simulink model "similinkProj"  (R2016a)
settings: Solver=VariableStepAuto  StartTime=0.0  StopTime=5  RelTol=1e-3
settings Model: Creator=bmcilw1  LastModifiedBy=bmcilw1

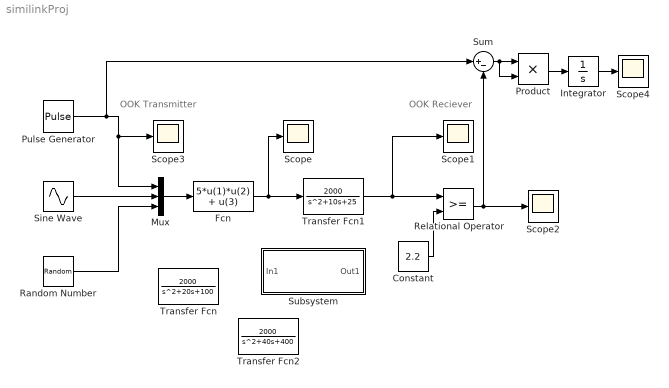
== system similinkProj ==
  note: OOK Transmitter
  note: OOK Reciever
  Constant : Constant  Value=2.2
  Fcn : Fcn  Expr=5*u(1)*u(2) + u(3)
  Integrator : Integrator
  Mux : Mux  Inputs=3
  Product : Product
  Pulse Generator : DiscretePulseGenerator  PulseType=Time based  PulseWidth=10  PhaseDelay=.2
  Random Number : RandomNumber  Variance=.25  SampleTime=0.001
  Relational Operator : RelationalOperator  OutDataTypeStr=boolean
  Scope{,1..4} (5 alike) : Scope
  Sine Wave : Sin  Amplitude=3  Frequency=50*2*pi  SampleTime=0.001
  Subsystem : Subsystem
  Sum : Sum  Inputs=|+-
  Transfer Fcn : TransferFcn  Numerator=[2000]  Denominator=[1 20 100]
  Transfer Fcn1 : TransferFcn  Numerator=[2000]  Denominator=[1 10 25]
  Transfer Fcn2 : TransferFcn  Numerator=[2000]  Denominator=[1 40 400]
  wires:
  Mux/1 -> Fcn/1
  Pulse Generator/1 -> Sum/1, Scope3/1, Mux/1
  Sine Wave/1 -> Mux/2
  Random Number/1 -> Mux/3
  Constant/1 -> Relational Operator/2
  Relational Operator/1 -> Scope2/1, Sum/2
  Fcn/1 -> Transfer Fcn1/1, Scope/1
  Product/1 -> Integrator/1
  Sum/1 -> Product/2, Product/1
  Integrator/1 -> Scope4/1
  Transfer Fcn1/1 -> Scope1/1, Relational Operator/1

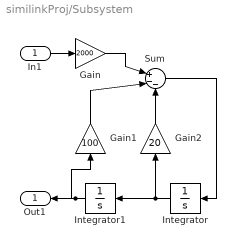
== system similinkProj/Subsystem ==
  In1 : Inport
  Gain : Gain  Gain=2000
  Gain1 : Gain  Gain=100
  Gain2 : Gain  Gain=20
  Integrator : Integrator
  Integrator1 : Integrator
  Sum : Sum  Inputs=|+--
  Out1 : Outport
  wires:
  Sum/1 -> Integrator/1
  Integrator/1 -> Gain2/1, Integrator1/1
  Gain2/1 -> Sum/3
  Integrator1/1 -> Gain1/1, Out1/1
  Gain1/1 -> Sum/2
  Gain/1 -> Sum/1
  In1/1 -> Gain/1
